simulink library "INT_CoEng_Stop"  (R2016b)
settings: Solver=VariableStepAuto  StartTime=0.0  StopTime=10.0  RelTol=1e-3
settings Model: Creator=Administrator  LastModifiedBy=Administrator

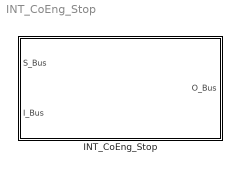
== system INT_CoEng_Stop ==
  INT_CoEng_Stop : Subsystem

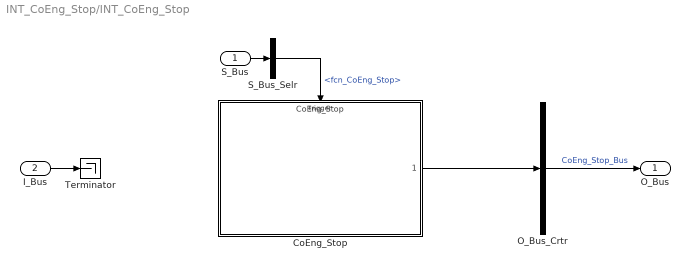
== system INT_CoEng_Stop/INT_CoEng_Stop ==
  S_Bus : Inport
  I_Bus : Inport  Port=2
  CoEng_Stop : ModelReference  ModelNameDialog=CoEng_Stop  SimulationMode=Normal  ModelReferenceVersion=1.2  TriggerPortName=function  TriggerPortTriggerType=function-call  TriggerPortStatesWhenEnabling=held
  O_Bus_Crtr : BusCreator  Inputs=1
  S_Bus_Selr : BusSelector  OutputSignals=fcn_CoEng_Stop
  Terminator : Terminator
  O_Bus : Outport
  wires:
  S_Bus_Selr/1 -> CoEng_Stop/Trigger  "<fcn_CoEng_Stop>"
  S_Bus/1 -> S_Bus_Selr/1
  I_Bus/1 -> Terminator/1
  O_Bus_Crtr/1 -> O_Bus/1  "CoEng_Stop_Bus"
  CoEng_Stop/1 -> O_Bus_Crtr/1
